simulink model "tp354182"  (Simulink 3.0)
settings: Solver=ode1  SolverMode=SingleTasking  StartTime=0.0  StopTime=t_sim  FixedStep=Ts  RelTol=1e-3
values from neighbouring files (symbols this model uses):
  D = exp(-Ts/Ta)    [init_I0_disc2.m]    (also in init_PID.m = input('Put D gain of controller (0)   = '); step_resp1.mat = 0.513417119033)
  I = input('Put I gain of controller (0.25) = ')    [init_PID.m]    (also in step_resp1.mat = 0.5)
  P = -alfa/Ks    [init_PI1_windupless.m]    (also in init_PID.m = input('Put P gain of controller (5)   = '); step_resp1.mat = 2)
  Ts = 0.2    [init_I0_disc2.m]    (also in init_PI0_windupless.m = 0.5; init_PI1_windupless.m; init_PID.m; step_resp1.mat)
  Umax = 5    [init_I0_disc2.m]    (also in init_PI0_windupless.m; init_PI1_windupless.m; init_PID.m; step_resp1.mat)
  Umin = 0    [init_I0_disc2.m]    (also in init_PI0_windupless.m; init_PI1_windupless.m; init_PID.m; step_resp1.mat)
libraries: simulink x1, udaq28LT_lib x1
settings Model: LastModifiedBy=mato  SaveFormat=Matrix  BooleanDataType=on

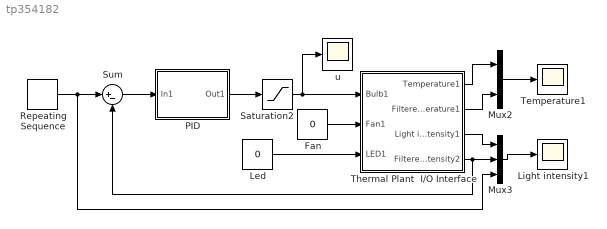
== system tp354182 ==
  Fan : Constant  Value=0
  Led : Constant  Value=0
  Light intensity1 : Scope
      settings: TickLabels=on  TimeRange=30  YMin=0  YMax=100  SaveName=yl  DataFormat=Matrix
  Mux2 : Mux  Inputs=2
  Mux3 : Mux  Inputs=3
  PID : Subsystem
  Repeating Sequence : simulink/Sources/Repeating Sequence  rep_seq_t=[0 60 60+Ts 120]  rep_seq_y=[20 20 40 40]
  Saturation2 : Saturate  UpperLimit=Umax  LowerLimit=Umin
  Sum : Sum  Inputs=|+-  SaturateOnIntegerOverflow=on
  Temperature1 : Scope
      settings: TickLabels=on  TimeRange=30  YMin=15  YMax=50  SaveName=yt  DataFormat=Matrix
  Thermal Plant  I/O Interface : Subsystem
      mask Display: disp('Thermo-optical\nPlant\nI/O Interface')
  u : Scope
      settings: TimeRange=120  YMin=-0.5  YMax=5.5  SaveName=u  DataFormat=Matrix  Decimation=10  SampleInput=on  SampleTime=Ts
  wires:
  Saturation2/1 -> u/1, Thermal Plant  I/O Interface/1(Bulb1)
  Sum/1 -> PID/1(In1)
  PID/1(Out1) -> Saturation2/1
  Repeating Sequence/1 -> Sum/1, Mux3/3
  Mux2/1 -> Temperature1/1
  Mux3/1 -> Light intensity1/1
  Fan/1 -> Thermal Plant  I/O Interface/2(Fan1)
  Led/1 -> Thermal Plant  I/O Interface/3(LED1)
  Thermal Plant  I/O Interface/1(Temperature1) -> Mux2/1
  Thermal Plant  I/O Interface/2(Filtered  temperature1) -> Mux2/2
  Thermal Plant  I/O Interface/3(Light intensity1) -> Mux3/1
  Thermal Plant  I/O Interface/4(Filtered  light intensity2) -> Mux3/2, Sum/2

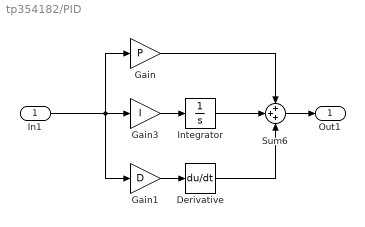
== system tp354182/PID ==
  In1 : Inport  Port=1  PortWidth=-1  SampleTime=-1  DataType=auto
      settings: SignalType=auto
  Derivative : Derivative
  Gain : Gain  Gain=P  SaturateOnIntegerOverflow=on
  Gain1 : Gain  Gain=D  SaturateOnIntegerOverflow=on
  Gain3 : Gain  Gain=I  SaturateOnIntegerOverflow=on
  Integrator : Integrator  ExternalReset=none  InitialConditionSource=internal  InitialCondition=0  LimitOutput=off  UpperSaturationLimit=inf  LowerSaturationLimit=-inf  ShowSaturationPort=off  ShowStatePort=off  AbsoluteTolerance=auto
  Sum6 : Sum  Inputs=+++  SaturateOnIntegerOverflow=on
  Out1 : Outport  Port=1
  wires:
  Gain3/1 -> Integrator/1
  Sum6/1 -> Out1/1
  In1/1 -> Gain/1, Gain3/1, Gain1/1
  Integrator/1 -> Sum6/2
  Gain/1 -> Sum6/1
  Gain1/1 -> Derivative/1
  Derivative/1 -> Sum6/3

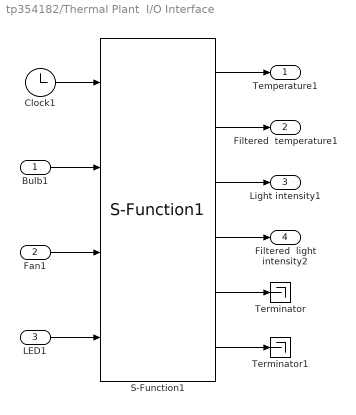
== system tp354182/Thermal Plant  I/O Interface ==
  Bulb1 : Inport  Port=1  PortWidth=-1  SampleTime=-1  DataType=auto
      settings: SignalType=auto
  Fan1 : Inport  Port=2  PortWidth=-1  SampleTime=-1  DataType=auto
      settings: SignalType=auto
  LED1 : Inport  Port=3  PortWidth=-1  SampleTime=-1  DataType=auto
      settings: SignalType=auto
  Clock1 : Clock
      settings: DisplayTime=off  Decimation=10
  S-Function1 : udaq28LT_lib/S-Function1  Priority=1  com_port=COM3  Ts=Ts  events_ot=2  rd_timeout=Ts/2*1000  matlab_prior=ABOVE_NORMAL_PRIORITY  warning=on  printout=off
  Terminator : Terminator
  Terminator1 : Terminator
  Temperature1 : Outport  Port=1
  Filtered  temperature1 : Outport  Port=2
  Light intensity1 : Outport  Port=3
  Filtered  light intensity2 : Outport  Port=4
  wires:
  S-Function1/1 -> Temperature1/1
  S-Function1/2 -> Filtered  temperature1/1
  Clock1/1 -> S-Function1/1
  Bulb1/1 -> S-Function1/2
  Fan1/1 -> S-Function1/3
  S-Function1/3 -> Light intensity1/1
  S-Function1/4 -> Filtered  light intensity2/1
  S-Function1/5 -> Terminator/1
  S-Function1/6 -> Terminator1/1
  LED1/1 -> S-Function1/4
